simulink model "APF_SMC"  (R2019a)
settings: Solver=FixedStepDiscrete  StartTime=0.0  StopTime=60  FixedStep=0.1  RelTol=1e-3
undefined symbols (not defined in the file): Kd_psi, Kd_Vx, Ki_psi, Ki_Vx, Kp_psi, Kp_Vx
libraries: simulink x8
settings Model: Creator=PC  LastModifiedBy=administrator
settings OptimizationCC: EnhancedBackFolding=on  PassReuseOutputArgsAs=Individual arguments  OptimizeBlockOrder=speed  DifferentSizesBufferReuse=on  OptimizationCustomize=off
settings DebuggingCC: ParameterTunabilityLossMsg=error
settings HardwareCC: ProdBitPerPointer=32  ProdBitPerSizeT=32  ProdBitPerPtrDiffT=32  ProdLargestAtomicInteger=Long  ProdLargestAtomicFloat=Double  ProdWordSize=32  ProdHWDeviceType=ARM Compatible->ARM Cortex
settings SFSimCC: MATLABDynamicMemAlloc=off
settings RTWCC: SystemTargetFile=ert.tlc  GenCodeOnly=on  TemplateMakefile=ert_default_tmf  GenerateReport=on  IncludeHyperlinkInReport=on  LaunchReport=on  TargetLang=C++  GenerateTraceInfo=on  GenerateTraceReport=on  GenerateTraceReportSl=on  GenerateTraceReportSf=on  GenerateTraceReportEml=on
settings CodeAppCC: ForceParamTrailComments=on  IgnoreCustomStorageClasses=off  OperatorAnnotations=on  SimulinkDataObjDesc=on  SFDataObjDesc=on  InsertBlockDesc=on
settings ERTTargetCC: TargetLangStandard=C++03 (ISO)  GenerateSampleERTMain=on  MultiInstanceERTCode=on  CodeInterfacePackaging=Reusable function  RootIOFormat=Structure reference  ERTCustomFileTemplate=example_file_process.tlc

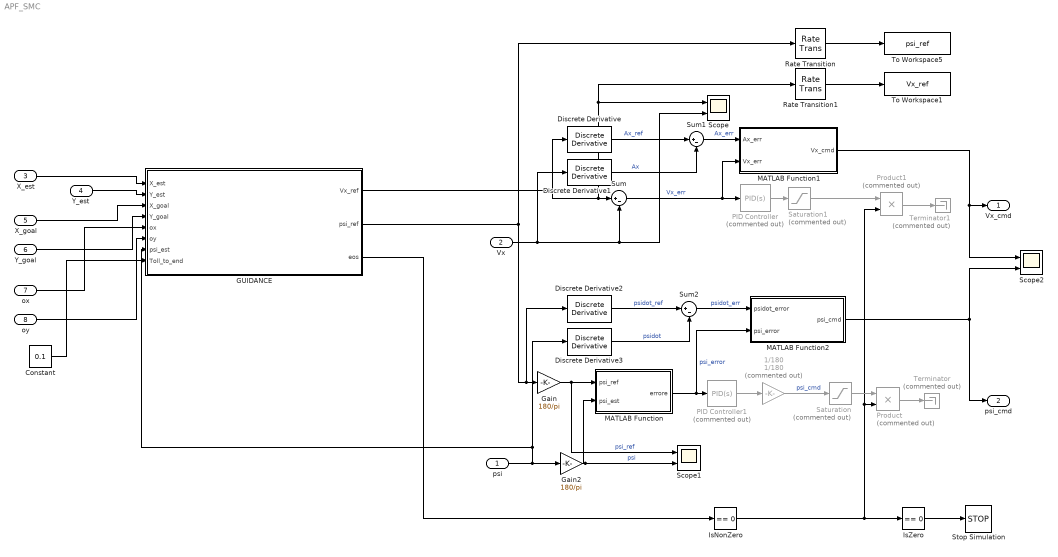
== system APF_SMC ==
  psi : Inport
  Vx : Inport  Port=2
  X_est : Inport  Port=3
  Y_est : Inport  Port=4
  X_goal : Inport  Port=5
  Y_goal : Inport  Port=6
  ox : Inport  Port=7
  oy : Inport  Port=8
  1/180 : Gain  Commented=on  Gain=1/180
  Constant : Constant  Value=0.1
  Discrete Derivative{,1..3} (4 alike) : simulink/Discrete/Discrete Derivative  gainval=1.0  ICPrevScaledInput=0.0  OutMin=[]  OutMax=[]  OutDataType=fixdt(1, 16)  OutScaling=2^-10  DoSatur=off
  "GUIDANCE " : Subsystem
  Gain : Gain  Gain=180/pi
  Gain2 : Gain  Gain=180/pi
  IsNonZero : simulink/Logic and Bit Operations/Compare To Zero  relop===  OutDataTypeStr=boolean
  IsZero : simulink/Logic and Bit Operations/Compare To Zero  relop===  OutDataTypeStr=boolean
  MATLAB Function : MATLAB Function  TreatAsAtomicUnit=on
  MATLAB Function1 : MATLAB Function  TreatAsAtomicUnit=on
  MATLAB Function2 : MATLAB Function  TreatAsAtomicUnit=on
  PID Controller : simulink/Continuous/PID Controller  Commented=on  Controller=PID  Form=Parallel  TimeDomain=Continuous-time  SampleTime=-1  IntegratorMethod=Forward Euler  FilterMethod=Forward Euler  ControllerParametersSource=internal  P=Kp_Vx  I=Ki_Vx  D=Kd_Vx  UseFilter=on  N=100  TunerSelectOption=Transfer Function Based (PID Tuner App)  InitialConditionSource=internal  InitialConditionForIntegrator=0  InitialConditionForFilter=0  DifferentiatorICPrevScaledInput=0  ExternalReset=none  TrackingMode=off  Kt=1  LimitOutput=off  UpperSaturationLimit=inf  LowerSaturationLimit=-inf  LinearizeAsGain=on  AntiWindupMode=none  Kb=1  POutMin=[]  POutMax=[]  IOutMin=[]  IOutMax=[]  DOutMin=[]  DOutMax=[]  NOutMin=[]  NOutMax=[]  SumOutMin=[]  SumOutMax=[]  SaturationOutMin=[]  SaturationOutMax=[]  PParamMin=[]  PParamMax=[]  IParamMin=[]  IParamMax=[]  DParamMin=[]  DParamMax=[]  NParamMin=[]  NParamMax=[]  KbParamMin=[]  KbParamMax=[]  KtParamMin=[]  KtParamMax=[]  KbOutMin=[]  KbOutMax=[]  KtOutMin=[]  KtOutMax=[]  IntegratorOutMin=[]  IntegratorOutMax=[]  FilterOutMin=[]  FilterOutMax=[]  SumI1OutMin=[]  SumI1OutMax=[]  SumI2OutMin=[]  SumI2OutMax=[]  SumI3OutMin=[]  SumI3OutMax=[]  SumI4OutMin=[]  SumI4OutMax=[]  SumDOutMin=[]  SumDOutMax=[]  DifferentiatorOutMin=[]  DifferentiatorOutMax=[]  FilterDiffOutCoefMin=[]  FilterDiffOutCoefMax=[]  ReciprocalOutMin=[]  ReciprocalOutMax=[]  SumDenOutMin=[]  SumDenOutMax=[]  SumNumOutMin=[]  SumNumOutMax=[]  DivideOutMin=[]  DivideOutMax=[]  IntegratorContinuousStateAttributes=''  IntegratorStateMustResolveToSignalObject=off  IntegratorRTWStateStorageClass=Auto  FilterContinuousStateAttributes=''  FilterStateMustResolveToSignalObject=off  FilterRTWStateStorageClass=Auto  ParallelPVariant=InternalParameters  IdealPVariant=Disabled  IVariant=InternalParameters  DVariant=InternalParameters  IntegratorVariant=Continuous  SatVariant=Disabled  AWVariant=Passthrough  PCopyVariant=Disabled  TRVariant=Disabled  FdbkBlocksVariant=Forward  IdealPFdbkVariant=Disabled  SatFdbkVariant=Disabled  DerivativeFilterVariant=ContFilter  NVariant=InternalParameters  NCopyVariant=Disabled  FilterICVariant=InternalICsFilter  IntegratorICVariant=InternalICs  ExternalResetVariant=Disabled  TRSumVariant=Passthrough  SumFdbkVariant=Disabled  SumVariant=Sum_PID
  PID Controller1 : simulink/Continuous/PID Controller  Commented=on  Controller=PID  Form=Parallel  TimeDomain=Continuous-time  SampleTime=-1  IntegratorMethod=Forward Euler  FilterMethod=Forward Euler  ControllerParametersSource=internal  P=Kp_psi  I=Ki_psi  D=Kd_psi  UseFilter=on  N=100  TunerSelectOption=Transfer Function Based (PID Tuner App)  InitialConditionSource=internal  InitialConditionForIntegrator=0  InitialConditionForFilter=0  DifferentiatorICPrevScaledInput=0  ExternalReset=none  TrackingMode=off  Kt=1  LimitOutput=off  UpperSaturationLimit=inf  LowerSaturationLimit=-inf  LinearizeAsGain=on  AntiWindupMode=none  Kb=1  POutMin=[]  POutMax=[]  IOutMin=[]  IOutMax=[]  DOutMin=[]  DOutMax=[]  NOutMin=[]  NOutMax=[]  SumOutMin=[]  SumOutMax=[]  SaturationOutMin=[]  SaturationOutMax=[]  PParamMin=[]  PParamMax=[]  IParamMin=[]  IParamMax=[]  DParamMin=[]  DParamMax=[]  NParamMin=[]  NParamMax=[]  KbParamMin=[]  KbParamMax=[]  KtParamMin=[]  KtParamMax=[]  KbOutMin=[]  KbOutMax=[]  KtOutMin=[]  KtOutMax=[]  IntegratorOutMin=[]  IntegratorOutMax=[]  FilterOutMin=[]  FilterOutMax=[]  SumI1OutMin=[]  SumI1OutMax=[]  SumI2OutMin=[]  SumI2OutMax=[]  SumI3OutMin=[]  SumI3OutMax=[]  SumI4OutMin=[]  SumI4OutMax=[]  SumDOutMin=[]  SumDOutMax=[]  DifferentiatorOutMin=[]  DifferentiatorOutMax=[]  FilterDiffOutCoefMin=[]  FilterDiffOutCoefMax=[]  ReciprocalOutMin=[]  ReciprocalOutMax=[]  SumDenOutMin=[]  SumDenOutMax=[]  SumNumOutMin=[]  SumNumOutMax=[]  DivideOutMin=[]  DivideOutMax=[]  IntegratorContinuousStateAttributes=''  IntegratorStateMustResolveToSignalObject=off  IntegratorRTWStateStorageClass=Auto  FilterContinuousStateAttributes=''  FilterStateMustResolveToSignalObject=off  FilterRTWStateStorageClass=Auto  ParallelPVariant=InternalParameters  IdealPVariant=Disabled  IVariant=InternalParameters  DVariant=InternalParameters  IntegratorVariant=Continuous  SatVariant=Disabled  AWVariant=Passthrough  PCopyVariant=Disabled  TRVariant=Disabled  FdbkBlocksVariant=Forward  IdealPFdbkVariant=Disabled  SatFdbkVariant=Disabled  DerivativeFilterVariant=ContFilter  NVariant=InternalParameters  NCopyVariant=Disabled  FilterICVariant=InternalICsFilter  IntegratorICVariant=InternalICs  ExternalResetVariant=Disabled  TRSumVariant=Passthrough  SumFdbkVariant=Disabled  SumVariant=Sum_PID
  Product : Product  Commented=on
  Product1 : Product  Commented=on
  Rate Transition : RateTransition
  Rate Transition1 : RateTransition
  Saturation : Saturate  Commented=on
  Saturation1 : Saturate  Commented=on  UpperLimit=1  LowerLimit=-1
  Scope : Scope  NumInputPorts=2
  Scope1 : Scope  NumInputPorts=2
  Scope2 : Scope  NumInputPorts=2
  Stop Simulation : Stop
  Sum : Sum  Inputs=|+-
  Sum1 : Sum  Inputs=|+-
  Sum2 : Sum  Inputs=|+-
  Terminator : Terminator  Commented=on
  Terminator1 : Terminator  Commented=on
  To Workspace1 : ToWorkspace  VariableName=Vx_ref  SaveFormat=Structure With Time  SampleTime=-1
  To Workspace5 : ToWorkspace  VariableName=psi_ref  SaveFormat=Structure With Time  SampleTime=-1
  Vx_cmd : Outport  VectorParamsAs1DForOutWhenUnconnected=on
  psi_cmd : Outport  Port=2  VectorParamsAs1DForOutWhenUnconnected=on
  wires:
  Gain/1 -> Scope1/1, MATLAB Function/1(psi_ref)  "psi_ref"
  Gain2/1 -> Scope1/2, MATLAB Function/2(psi_est)  "psi"
  "GUIDANCE "/3(eos) -> IsNonZero/1
  1/180/1 -> Saturation/1  "psi_cmd"
  Discrete Derivative2/1 -> Sum2/1  "psidot_ref"
  Product1/1 -> Terminator1/1
  Product/1 -> Terminator/1
  IsNonZero/1 -> IsZero/1, Product1/2, Product/2
  Sum2/1 -> MATLAB Function2/1(psidot_error)  "psidot_err"
  X_goal/1 -> "GUIDANCE "/3(X_goal)
  MATLAB Function2/1(psi_cmd) -> psi_cmd/1, Scope2/2
  IsZero/1 -> Stop Simulation/1
  Constant/1 -> "GUIDANCE "/8(Toll_to_end)
  Discrete Derivative3/1 -> Sum2/2  "psidot"
  Rate Transition/1 -> To Workspace5/1
  Y_est/1 -> "GUIDANCE "/2(Y_est)
  Saturation1/1 -> Product1/1
  X_est/1 -> "GUIDANCE "/1(X_est)
  MATLAB Function/1(errore) -> PID Controller1/1, MATLAB Function2/2(psi_error)  "psi_error"
  PID Controller/1 -> Saturation1/1
  ox/1 -> "GUIDANCE "/5(ox)
  oy/1 -> "GUIDANCE "/6(oy)
  Sum/1 -> PID Controller/1, MATLAB Function1/2(Vx_err)  "Vx_err"
  MATLAB Function1/1(Vx_cmd) -> Scope2/1, Vx_cmd/1
  Saturation/1 -> Product/1
  Discrete Derivative1/1 -> Sum1/2  "Ax"
  "GUIDANCE "/1(Vx_ref) -> Rate Transition1/1, Scope/1, Sum/1, Discrete Derivative/1
  Y_goal/1 -> "GUIDANCE "/4(Y_goal)
  PID Controller1/1 -> 1/180/1
  Vx/1 -> Scope/2, Sum/2, Discrete Derivative1/1
  Discrete Derivative/1 -> Sum1/1  "Ax_ref"
  Rate Transition1/1 -> To Workspace1/1
  Sum1/1 -> MATLAB Function1/1(Ax_err)  "Ax_err"
  psi/1 -> "GUIDANCE "/7(psi_est), Discrete Derivative3/1, Gain2/1
  "GUIDANCE "/2(psi_ref) -> Discrete Derivative2/1, Gain/1, Rate Transition/1

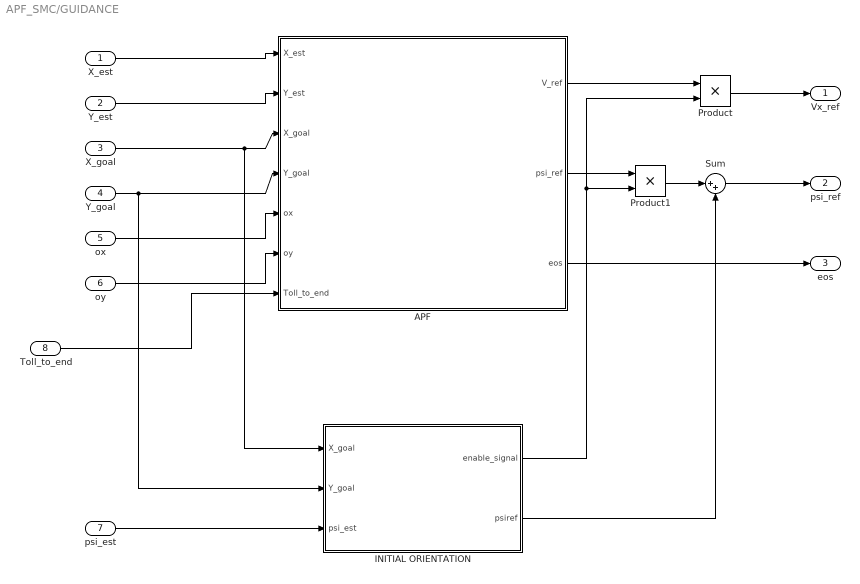
== system APF_SMC/GUIDANCE  ==
  X_est : Inport
  Y_est : Inport  Port=2
  X_goal : Inport  Port=3
  Y_goal : Inport  Port=4
  ox : Inport  Port=5
  oy : Inport  Port=6
  psi_est : Inport  Port=7
  Toll_to_end : Inport  Port=8
  APF : Subsystem
  INITIAL ORIENTATION : Subsystem
  Product : Product
  Product1 : Product
  Sum : Sum  Inputs=|++
  Vx_ref : Outport  VectorParamsAs1DForOutWhenUnconnected=on
  psi_ref : Outport  Port=2  VectorParamsAs1DForOutWhenUnconnected=on
  eos : Outport  Port=3  VectorParamsAs1DForOutWhenUnconnected=on
  wires:
  X_goal/1 -> INITIAL ORIENTATION/1(X_goal), APF/3(X_goal)
  Y_goal/1 -> INITIAL ORIENTATION/2(Y_goal), APF/4(Y_goal)
  X_est/1 -> APF/1(X_est)
  Y_est/1 -> APF/2(Y_est)
  ox/1 -> APF/5(ox)
  oy/1 -> APF/6(oy)
  Sum/1 -> psi_ref/1
  psi_est/1 -> INITIAL ORIENTATION/3(psi_est)
  INITIAL ORIENTATION/2(psiref) -> Sum/2
  APF/1(V_ref) -> Product/1
  Product/1 -> Vx_ref/1
  INITIAL ORIENTATION/1(enable_signal) -> Product1/2, Product/2
  APF/2(psi_ref) -> Product1/1
  Product1/1 -> Sum/1
  APF/3(eos) -> eos/1
  Toll_to_end/1 -> APF/7(Toll_to_end)

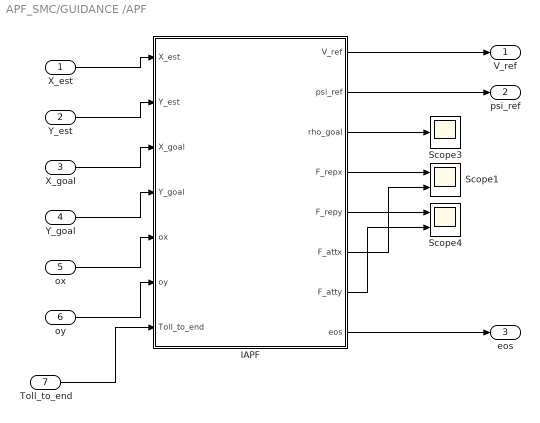
== system APF_SMC/GUIDANCE /APF ==
  X_est : Inport
  Y_est : Inport  Port=2
  X_goal : Inport  Port=3
  Y_goal : Inport  Port=4
  ox : Inport  Port=5
  oy : Inport  Port=6
  Toll_to_end : Inport  Port=7
  IAPF : MATLAB Function  TreatAsAtomicUnit=on
  Scope1 : Scope  NumInputPorts=2
  Scope3 : Scope
  Scope4 : Scope  NumInputPorts=2
  V_ref : Outport  VectorParamsAs1DForOutWhenUnconnected=on
  psi_ref : Outport  Port=2  VectorParamsAs1DForOutWhenUnconnected=on
  eos : Outport  Port=3  VectorParamsAs1DForOutWhenUnconnected=on
  wires:
  IAPF/1(V_ref) -> V_ref/1
  IAPF/6(F_attx) -> Scope1/2
  IAPF/3(rho_goal) -> Scope3/1
  IAPF/4(F_repx) -> Scope1/1
  IAPF/7(F_atty) -> Scope4/2
  IAPF/5(F_repy) -> Scope4/1
  X_est/1 -> IAPF/1(X_est)
  ox/1 -> IAPF/5(ox)
  IAPF/2(psi_ref) -> psi_ref/1
  Y_est/1 -> IAPF/2(Y_est)
  oy/1 -> IAPF/6(oy)
  IAPF/8(eos) -> eos/1
  X_goal/1 -> IAPF/3(X_goal)
  Y_goal/1 -> IAPF/4(Y_goal)
  Toll_to_end/1 -> IAPF/7(Toll_to_end)

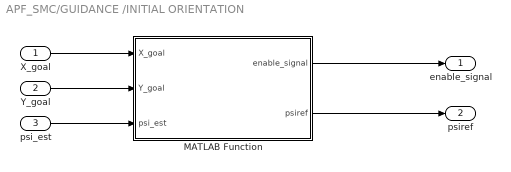
== system APF_SMC/GUIDANCE /INITIAL ORIENTATION ==
  X_goal : Inport
  Y_goal : Inport  Port=2
  psi_est : Inport  Port=3
  MATLAB Function : MATLAB Function  TreatAsAtomicUnit=on
  enable_signal : Outport  VectorParamsAs1DForOutWhenUnconnected=on
  psiref : Outport  Port=2  VectorParamsAs1DForOutWhenUnconnected=on
  wires:
  psi_est/1 -> MATLAB Function/3(psi_est)
  MATLAB Function/2(psiref) -> psiref/1
  Y_goal/1 -> MATLAB Function/2(Y_goal)
  X_goal/1 -> MATLAB Function/1(X_goal)
  MATLAB Function/1(enable_signal) -> enable_signal/1

== matlab function APF_SMC/GUIDANCE /INITIAL ORIENTATION/MATLAB Function ==
  data: X_goal input; enable_signal output; Y_goal input; psi_est input; psiref output
function [enable_signal, psiref] = fcn(X_goal, Y_goal, psi_est)
psiref=0;
enable_signal=0;

persistent en
if isempty(en)
    en=0;
end

if en==0
if -pi<psi_est && psi_est<=-pi/2 
  if X_goal>=0 && Y_goal>=0
      enable_signal=0;
      psiref=0;
      en=0;
  end
   if X_goal>0 && Y_goal<0
      enable_signal=0;
      psiref=0;
      en=0;
   end
    if X_goal<=0 && Y_goal<=0
      enable_signal=1;
      en=1;
      psiref=0;
    end
    if X_goal<0 && Y_goal>0
      enable_signal=1;
      en=1;
      psiref=0;
    end
end
if pi/2<psi_est && psi_est<=pi 
  if X_goal>=0 && Y_goal>=0
      enable_signal=0;
      psiref=0;
      en=0;
  end
   if X_goal>0 && Y_goal<0
      enable_signal=0;
      psiref=0;
      en=0;
   end
    if X_goal<=0 && Y_goal<=0
      enable_signal=1;
      en=1;
      psiref=0;
    end
    if X_goal<0 && Y_goal>0
      enable_signal=1;
      en=1;
      psiref=0;
    end
end

if -pi/2<=psi_est && psi_est<=pi/2
  if X_goal>=0 && Y_goal>=0
      enable_signal=1;
      en=1;
      psiref=0;
  end
   if X_goal>0 && Y_goal<0
      enable_signal=1;
      en=1;
      psiref=0;
   end
    if X_goal<=0 && Y_goal<=0
      enable_signal=0;
      psiref=-pi;
      en=0;
    end
    if X_goal<0 && Y_goal>0
      enable_signal=0;
      psiref=pi;
      en=0;
    end
end
else
    enable_signal=1;
    psiref=0;
end

== matlab function APF_SMC/MATLAB Function1 ==
  data: Ax_err input; Vx_cmd output; Vx_err input
function Vx_cmd = SMC_Vx(Ax_err, Vx_err)
% SMC params
lamda = 30;
K = 0.1;
% Sliding surface
s = zeros(1);
s = (Ax_err) + lamda*(Vx_err);


Vx_cmd = K*sign(s);

== matlab function APF_SMC/MATLAB Function ==
  data: psi_ref input; errore output; psi_est input
function errore = fcn(psi_ref, psi_est)
errore=psi_ref-psi_est;

if abs(errore)>180
    errore=errore-360*sign(errore);
end

== matlab function APF_SMC/GUIDANCE /APF/IAPF ==
  data: X_est input; V_ref output; Y_est input; X_goal input; Y_goal input; ox input; oy input; psi_ref output; rho_goal output; F_repx output; F_repy output; F_attx output; F_atty output; eos output; Toll_to_end input
function [V_ref, psi_ref, rho_goal, F_repx, F_repy, F_attx, F_atty, eos]  = fcn(X_est, Y_est, X_goal, Y_goal,  ox, oy, Toll_to_end)

% Potential field characteristics
rho_0=0.7;                   % Area of influence of obstacle  [m]
kp = 0.15;                   % Attractive pottential gain
eta = 0.05;                  % Repulsive potential gain

q=[X_est, Y_est]';           % Actual position [m]       
qg=[X_goal, Y_goal]';        % Goal position   [m]
rho_goal=norm(q-qg,2);       % Distance actual position-goal position
d=2;                         % Distance from goal, point of attractive field characteristic switching

% ATTRACTIVE
if rho_goal<=d
F_attx = -kp*(X_est-X_goal);
F_atty = -kp*(Y_est-Y_goal);
else    
F_attx = -kp*(X_est-X_goal)*d/rho_goal;
F_atty = -kp*(Y_est-Y_goal)*d/rho_goal;
end


% REPULSIVE
F_repx=0;
F_repy=0;
dmin=10000;
qc=[0 0]';
obst=0;

for k=1:length(ox)
    qc=[ox(k) oy(k)]';                          % Obstacle position [m]
    dq = norm(q-qc,2);                          % Distance actual position- obstacle position
     
    if dmin >= dq
        dmin = dq;
        min_ost = k;
        qc=[ox(min_ost) oy(min_ost)]';
        rho = norm(q-qc,2) ;                    % Distance with the nearest obstacle
        
        if rho<=rho_0                           % Inside obstacle area! Danger
           F_repx=eta*(1/rho - 1/rho_0)*1/(rho).^2*(X_est-ox(min_ost))/norm(q-qc,2);
           F_repy=eta*(1/rho - 1/rho_0)*1/(rho).^2*(Y_est-oy(min_ost))/norm(q-qc,2);  
           obst=1/rho;
        end
     
     end
end

% To find the goal if the obstacle is near
dob=0.3;
dgr=0.3;

if norm(qg-qc,2)<=dob && norm(q-qg,2)<=dgr
    F_totx=F_attx;
    F_toty=F_atty;
else
    F_totx = F_attx+F_repx;
    F_toty = F_atty+F_repy;
end

% Potential Force
F_tot=norm([F_totx,F_toty]);


% ORIENTATION REFERENCE SIGNAL
psi_ref=atan2(F_toty,F_totx);


% VELOCITY REFERENCE SIGNAL
% 1° prova per il campo di velocità
% V_ref=F_totx/F_tot*0.3;

% 2° prova per il campo di velocità
delta=0.4/rho_goal+obst;
V_ref= 0.3*2/(2+delta);

eos = 0;
% END OF SIMULATION
if abs(rho_goal)<=Toll_to_end
    eos=1;
end

% Mathematical minimum
if F_tot==0
    psi_ref=0;
    V_ref=-0.3;
end

== matlab function APF_SMC/MATLAB Function2 ==
  data: psidot_error input; psi_cmd output; psi_error input
function psi_cmd = SMC_psi(psidot_error, psi_error)
% SMC params
lamda = 100;
K = 0.2;
% Sliding surface
s = zeros(1);
s = (psidot_error) + lamda*(psi_error);


psi_cmd = K*sign(s);
